simulink model "fft_biplex_test3"  (Simulink 7.6)
settings: Solver=ode45  StartTime=0.0  StopTime=5000  RelTol=1e-3
libraries: xbsIndex_r4 x1382, casper_library x82, monroe_library x27, xps_library x17, dspsigops x16, simulink x1
(part 2 of 13)

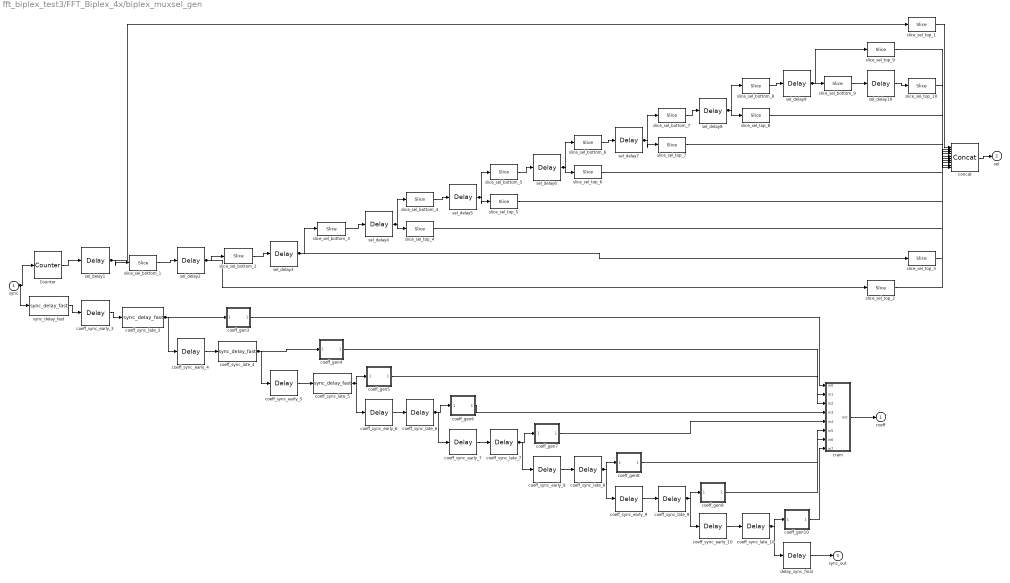
== system fft_biplex_test3/FFT_Biplex_4x/biplex_muxsel_gen ==
  sync : Inport
  Counter : xbsIndex_r4/Counter  cnt_type=Free Running  cnt_to=Inf  operation=Up  start_count=0  cnt_by_val=1  arith_type=Unsigned  n_bits=10  bin_pt=0  load_pin=off  rst=on  en=off  explicit_period=on  period=1  dbl_ovrd=off  use_behavioral_HDL=off  implementation=Fabric  block_type=counter
  coeff_gen10 : Subsystem
  coeff_gen3 : Subsystem
  coeff_gen4 : Subsystem
  coeff_gen5 : Subsystem
  coeff_gen6 : Subsystem
  coeff_gen7 : Subsystem
  coeff_gen8 : Subsystem
  coeff_gen9 : Subsystem
  coeff_sync_early_{4..10} (7 alike) : xbsIndex_r4/Delay  en=off  latency=8  dbl_ovrd=off  reg_retiming=off  block_type=delay
  coeff_sync_early_3 : xbsIndex_r4/Delay  en=off  latency=13  dbl_ovrd=off  reg_retiming=off  block_type=delay
  coeff_sync_late_10 : xbsIndex_r4/Delay  en=off  latency=1  dbl_ovrd=off  reg_retiming=off  block_type=delay
  coeff_sync_late_3 : monroe_library/sync_delay_fast  SystemSampleTime=-1  delay_len=128
  coeff_sync_late_4 : monroe_library/sync_delay_fast  SystemSampleTime=-1  delay_len=64
  coeff_sync_late_5 : monroe_library/sync_delay_fast  SystemSampleTime=-1  delay_len=32
  coeff_sync_late_6 : xbsIndex_r4/Delay  en=off  latency=16  dbl_ovrd=off  reg_retiming=off  block_type=delay
  coeff_sync_late_7 : xbsIndex_r4/Delay  en=off  latency=8  dbl_ovrd=off  reg_retiming=off  block_type=delay
  coeff_sync_late_8 : xbsIndex_r4/Delay  en=off  latency=4  dbl_ovrd=off  reg_retiming=off  block_type=delay
  coeff_sync_late_9 : xbsIndex_r4/Delay  en=off  latency=2  dbl_ovrd=off  reg_retiming=off  block_type=delay
  concat : xbsIndex_r4/Concat  num_inputs=10  dbl_ovrd=off  block_type=concat
  cram : Subsystem
  delay_sync_final : xbsIndex_r4/Delay  en=off  latency=6  dbl_ovrd=off  reg_retiming=off  block_type=delay
  sel_delay1 : xbsIndex_r4/Delay  en=off  latency=1  dbl_ovrd=off  reg_retiming=off  block_type=delay
  sel_delay{4..10} (7 alike) : xbsIndex_r4/Delay  en=off  latency=8  dbl_ovrd=off  reg_retiming=off  block_type=delay
  sel_delay2 : xbsIndex_r4/Delay  en=off  latency=4  dbl_ovrd=off  reg_retiming=off  block_type=delay
  sel_delay3 : xbsIndex_r4/Delay  en=off  latency=7  dbl_ovrd=off  reg_retiming=off  block_type=delay
  slice_sel_bottom_1 : xbsIndex_r4/Slice  nbits=9  boolean_output=off  mode=Lower Bit Location + Width  bit1=0  base1=LSB of Input  bit0=0  base0=LSB of Input  dbl_ovrd=off  block_type=slice
  slice_sel_bottom_2 : xbsIndex_r4/Slice  nbits=8  boolean_output=off  mode=Lower Bit Location + Width  bit1=0  base1=LSB of Input  bit0=0  base0=LSB of Input  dbl_ovrd=off  block_type=slice
  slice_sel_bottom_3 : xbsIndex_r4/Slice  nbits=7  boolean_output=off  mode=Lower Bit Location + Width  bit1=0  base1=LSB of Input  bit0=0  base0=LSB of Input  dbl_ovrd=off  block_type=slice
  slice_sel_bottom_4 : xbsIndex_r4/Slice  nbits=6  boolean_output=off  mode=Lower Bit Location + Width  bit1=0  base1=LSB of Input  bit0=0  base0=LSB of Input  dbl_ovrd=off  block_type=slice
  slice_sel_bottom_5 : xbsIndex_r4/Slice  nbits=5  boolean_output=off  mode=Lower Bit Location + Width  bit1=0  base1=LSB of Input  bit0=0  base0=LSB of Input  dbl_ovrd=off  block_type=slice
  slice_sel_bottom_6 : xbsIndex_r4/Slice  nbits=4  boolean_output=off  mode=Lower Bit Location + Width  bit1=0  base1=LSB of Input  bit0=0  base0=LSB of Input  dbl_ovrd=off  block_type=slice
  slice_sel_bottom_7 : xbsIndex_r4/Slice  nbits=3  boolean_output=off  mode=Lower Bit Location + Width  bit1=0  base1=LSB of Input  bit0=0  base0=LSB of Input  dbl_ovrd=off  block_type=slice
  slice_sel_bottom_8 : xbsIndex_r4/Slice  nbits=2  boolean_output=off  mode=Lower Bit Location + Width  bit1=0  base1=LSB of Input  bit0=0  base0=LSB of Input  dbl_ovrd=off  block_type=slice
  slice_sel_bottom_9 : xbsIndex_r4/Slice  nbits=1  boolean_output=off  mode=Lower Bit Location + Width  bit1=0  base1=LSB of Input  bit0=0  base0=LSB of Input  dbl_ovrd=off  block_type=slice
  slice_sel_top_{1..10} (10 alike) : xbsIndex_r4/Slice  nbits=1  boolean_output=on  mode=Upper Bit Location + Width  bit1=0  base1=MSB of Input  bit0=0  base0=MSB of Input  dbl_ovrd=off  block_type=slice
  sync_delay_fast : monroe_library/sync_delay_fast  SystemSampleTime=-1  delay_len=768
  coeff : Outport
  sel : Outport  Port=2
  sync_out : Outport  Port=3
  wires:
  sync_delay_fast/1 -> coeff_sync_early_3/1
  coeff_sync_early_3/1 -> coeff_sync_late_3/1
  coeff_sync_early_4/1 -> coeff_sync_late_4/1
  coeff_sync_early_5/1 -> coeff_sync_late_5/1
  coeff_sync_early_6/1 -> coeff_sync_late_6/1
  coeff_sync_early_7/1 -> coeff_sync_late_7/1
  coeff_sync_early_8/1 -> coeff_sync_late_8/1
  coeff_sync_early_9/1 -> coeff_sync_late_9/1
  coeff_sync_early_10/1 -> coeff_sync_late_10/1
  coeff_gen3/1(coeff) -> cram/1(in0)
  coeff_gen4/1(coeff) -> cram/2(in1)
  coeff_gen5/1(coeff) -> cram/3(in2)
  coeff_gen6/1(coeff) -> cram/4(in3)
  coeff_gen7/1(coeff) -> cram/5(in4)
  coeff_gen8/1(coeff) -> cram/6(in5)
  coeff_gen9/1(coeff) -> cram/7(in6)
  coeff_gen10/1(coeff) -> cram/8(in7)
  cram/1(out) -> coeff/1
  Counter/1 -> sel_delay1/1
  slice_sel_bottom_1/1 -> sel_delay2/1
  slice_sel_bottom_2/1 -> sel_delay3/1
  slice_sel_bottom_3/1 -> sel_delay4/1
  slice_sel_bottom_4/1 -> sel_delay5/1
  slice_sel_bottom_5/1 -> sel_delay6/1
  slice_sel_bottom_6/1 -> sel_delay7/1
  slice_sel_bottom_7/1 -> sel_delay8/1
  slice_sel_bottom_8/1 -> sel_delay9/1
  slice_sel_bottom_9/1 -> sel_delay10/1
  sel_delay10/1 -> slice_sel_top_10/1
  slice_sel_top_1/1 -> concat/1
  slice_sel_top_2/1 -> concat/2
  slice_sel_top_3/1 -> concat/3
  slice_sel_top_4/1 -> concat/4
  slice_sel_top_5/1 -> concat/5
  slice_sel_top_6/1 -> concat/6
  slice_sel_top_7/1 -> concat/7
  slice_sel_top_8/1 -> concat/8
  slice_sel_top_9/1 -> concat/9
  slice_sel_top_10/1 -> concat/10
  concat/1 -> sel/1
  delay_sync_final/1 -> sync_out/1
  sel_delay9/1 -> slice_sel_top_9/1, slice_sel_bottom_9/1
  sel_delay8/1 -> slice_sel_top_8/1, slice_sel_bottom_8/1
  sel_delay7/1 -> slice_sel_top_7/1, slice_sel_bottom_7/1
  sel_delay6/1 -> slice_sel_top_6/1, slice_sel_bottom_6/1
  sel_delay5/1 -> slice_sel_top_5/1, slice_sel_bottom_5/1
  sel_delay4/1 -> slice_sel_top_4/1, slice_sel_bottom_4/1
  sel_delay3/1 -> slice_sel_top_3/1, slice_sel_bottom_3/1
  sel_delay2/1 -> slice_sel_top_2/1, slice_sel_bottom_2/1
  sel_delay1/1 -> slice_sel_top_1/1, slice_sel_bottom_1/1
  coeff_sync_late_10/1 -> coeff_gen10/1(sync), delay_sync_final/1
  coeff_sync_late_9/1 -> coeff_gen9/1(sync), coeff_sync_early_10/1
  coeff_sync_late_8/1 -> coeff_gen8/1(sync), coeff_sync_early_9/1
  coeff_sync_late_7/1 -> coeff_gen7/1(sync), coeff_sync_early_8/1
  coeff_sync_late_6/1 -> coeff_gen6/1(sync), coeff_sync_early_7/1
  coeff_sync_late_5/1 -> coeff_gen5/1(sync), coeff_sync_early_6/1
  coeff_sync_late_4/1 -> coeff_gen4/1(sync), coeff_sync_early_5/1
  coeff_sync_late_3/1 -> coeff_gen3/1(sync), coeff_sync_early_4/1
  sync/1 -> sync_delay_fast/1, Counter/1

== system fft_biplex_test3/FFT_Biplex_4x/cram0 ==
  in0 : Inport
  in1 : Inport  Port=2
  concat : xbsIndex_r4/Concat  num_inputs=2  dbl_ovrd=off  block_type=concat
  reinterpret_1 : xbsIndex_r4/Reinterpret  force_arith_type=on  arith_type=Unsigned  force_bin_pt=on  bin_pt=0  block_type=reinterpret
      settings: infoedit="Changes signal type without altering the binary representation.   You can changed the signal between signed and unsigned, and relocate the binary point.<br><br>Hardware notes: In hardware this block costs nothing.<br><br>Example:  Suppose the input is 6 bits wide, signed, with 2 fractional bits, and the output is forced to unsigned with 0 fractional bits.  Then an input of -2.0 (1110.00 in binary 2's complement) becomes an output of 56 (111000 in binary)."
  reinterpret_2 : xbsIndex_r4/Reinterpret  force_arith_type=on  arith_type=Unsigned  force_bin_pt=on  bin_pt=0  block_type=reinterpret
      settings: infoedit="Changes signal type without altering the binary representation.   You can changed the signal between signed and unsigned, and relocate the binary point.<br><br>Hardware notes: In hardware this block costs nothing.<br><br>Example:  Suppose the input is 6 bits wide, signed, with 2 fractional bits, and the output is forced to unsigned with 0 fractional bits.  Then an input of -2.0 (1110.00 in binary 2's complement) becomes an output of 56 (111000 in binary)."
  out : Outport
  wires:
  in0/1 -> reinterpret_1/1
  in1/1 -> reinterpret_2/1
  reinterpret_1/1 -> concat/1
  reinterpret_2/1 -> concat/2
  concat/1 -> out/1

== system fft_biplex_test3/FFT_Biplex_4x/cram1 ==
  in0 : Inport
  in1 : Inport  Port=2
  concat : xbsIndex_r4/Concat  num_inputs=2  dbl_ovrd=off  block_type=concat
  reinterpret_1 : xbsIndex_r4/Reinterpret  force_arith_type=on  arith_type=Unsigned  force_bin_pt=on  bin_pt=0  block_type=reinterpret
      settings: infoedit="Changes signal type without altering the binary representation.   You can changed the signal between signed and unsigned, and relocate the binary point.<br><br>Hardware notes: In hardware this block costs nothing.<br><br>Example:  Suppose the input is 6 bits wide, signed, with 2 fractional bits, and the output is forced to unsigned with 0 fractional bits.  Then an input of -2.0 (1110.00 in binary 2's complement) becomes an output of 56 (111000 in binary)."
  reinterpret_2 : xbsIndex_r4/Reinterpret  force_arith_type=on  arith_type=Unsigned  force_bin_pt=on  bin_pt=0  block_type=reinterpret
      settings: infoedit="Changes signal type without altering the binary representation.   You can changed the signal between signed and unsigned, and relocate the binary point.<br><br>Hardware notes: In hardware this block costs nothing.<br><br>Example:  Suppose the input is 6 bits wide, signed, with 2 fractional bits, and the output is forced to unsigned with 0 fractional bits.  Then an input of -2.0 (1110.00 in binary 2's complement) becomes an output of 56 (111000 in binary)."
  out : Outport
  wires:
  in0/1 -> reinterpret_1/1
  in1/1 -> reinterpret_2/1
  reinterpret_1/1 -> concat/1
  reinterpret_2/1 -> concat/2
  concat/1 -> out/1

== system fft_biplex_test3/FFT_Biplex_4x/stage_1 ==
  a : Inport
  b : Inport  Port=2
  sync : Inport  Port=3
  mux_sel : Inport  Port=4
  Mux : xbsIndex_r4/Mux  inputs=2  en=off  latency=0  precision=Full  arith_type="Signed  (2's comp)"  n_bits=8  bin_pt=2  quantization=Truncate  overflow=Wrap  dbl_ovrd=off  block_type=mux
  Mux1 : xbsIndex_r4/Mux  inputs=2  en=off  latency=0  precision=Full  arith_type="Signed  (2's comp)"  n_bits=8  bin_pt=2  quantization=Truncate  overflow=Wrap  dbl_ovrd=off  block_type=mux
  delay_mid : xbsIndex_r4/Delay  en=off  latency=1  dbl_ovrd=off  reg_retiming=off  block_type=delay
  delay_mid1 : xbsIndex_r4/Delay  en=off  latency=1  dbl_ovrd=off  reg_retiming=off  block_type=delay
  delay_start : xbsIndex_r4/Delay  en=off  latency=1  dbl_ovrd=off  reg_retiming=off  block_type=delay
  delay_start1 : xbsIndex_r4/Delay  en=off  latency=1  dbl_ovrd=off  reg_retiming=off  block_type=delay
  double_delay_bram_fast : monroe_library/double_delay_bram_fast  SystemSampleTime=-1  delay_len=512  bram_latency=2  register_counter=0
  sync_delay_fast1 : monroe_library/sync_delay_fast  SystemSampleTime=-1  delay_len=512
  twiddle_stage1 : monroe_library/twiddle_stage1  SystemSampleTime=-1  input_bit_width=18  out_n_bits=18  downshift_at_end=1
  a+bw : Outport
  a-bw : Outport  Port=2
  sync_out : Outport  Port=3
  wires:
  Mux1/1 -> double_delay_bram_fast/1
  double_delay_bram_fast/1 -> delay_mid/1
  Mux/1 -> delay_mid1/1
  a/1 -> delay_start/1
  b/1 -> delay_start1/1
  delay_start1/1 -> double_delay_bram_fast/2
  sync/1 -> sync_delay_fast1/1
  delay_mid/1 -> twiddle_stage1/1
  delay_mid1/1 -> twiddle_stage1/2
  sync_delay_fast1/1 -> twiddle_stage1/3
  twiddle_stage1/1 -> a+bw/1
  twiddle_stage1/2 -> a-bw/1
  twiddle_stage1/3 -> sync_out/1
  delay_start/1 -> Mux/3, Mux1/2
  double_delay_bram_fast/2 -> Mux/2, Mux1/3
  mux_sel/1 -> Mux/1, Mux1/1

== system fft_biplex_test3/FFT_Biplex_4x/stage_10 ==
  a : Inport
  b : Inport  Port=2
  sync : Inport  Port=3
  coeff : Inport  Port=4
  mux_sel : Inport  Port=5
  Mux : xbsIndex_r4/Mux  inputs=2  en=off  latency=0  precision=Full  arith_type="Signed  (2's comp)"  n_bits=8  bin_pt=2  quantization=Truncate  overflow=Wrap  dbl_ovrd=off  block_type=mux
  Mux1 : xbsIndex_r4/Mux  inputs=2  en=off  latency=0  precision=Full  arith_type="Signed  (2's comp)"  n_bits=8  bin_pt=2  quantization=Truncate  overflow=Wrap  dbl_ovrd=off  block_type=mux
  delay_ddbf_1 : xbsIndex_r4/Delay  en=off  latency=1  dbl_ovrd=off  reg_retiming=off  block_type=delay
  delay_ddbf_2 : xbsIndex_r4/Delay  en=off  latency=1  dbl_ovrd=off  reg_retiming=off  block_type=delay
  delay_end : xbsIndex_r4/Delay  en=off  latency=2  dbl_ovrd=off  reg_retiming=off  block_type=delay
  delay_mid : xbsIndex_r4/Delay  en=off  latency=2  dbl_ovrd=off  reg_retiming=off  block_type=delay
  delay_mid1 : xbsIndex_r4/Delay  en=off  latency=1  dbl_ovrd=off  reg_retiming=off  block_type=delay
  delay_start : xbsIndex_r4/Delay  en=off  latency=1  dbl_ovrd=off  reg_retiming=off  block_type=delay
  delay_start1 : xbsIndex_r4/Delay  en=off  latency=1  dbl_ovrd=off  reg_retiming=off  block_type=delay
  sync_delay : xbsIndex_r4/Delay  en=off  latency=1  dbl_ovrd=off  reg_retiming=off  block_type=delay
  twiddle_cheap : monroe_library/twiddle_cheap  SystemSampleTime=-1  a_n_bits=18  a_bin_pt=17  b_n_bits=18  b_bin_pt=17  w_n_bits=18  w_bin_pt=17  a_delay=0  apbw_delay=0  out_n_bits=18  downshift_at_end=1
  a+bw : Outport
  a-bw : Outport  Port=2
  sync_out : Outport  Port=3
  wires:
  Mux1/1 -> delay_ddbf_1/1
  delay_end/1 -> a+bw/1
  delay_ddbf_1/1 -> delay_mid/1
  Mux/1 -> delay_mid1/1
  a/1 -> delay_start/1
  b/1 -> delay_start1/1
  delay_start1/1 -> delay_ddbf_2/1
  sync/1 -> sync_delay/1
  delay_mid/1 -> twiddle_cheap/1
  delay_mid1/1 -> twiddle_cheap/2
  coeff/1 -> twiddle_cheap/3
  sync_delay/1 -> twiddle_cheap/4
  twiddle_cheap/1 -> delay_end/1
  twiddle_cheap/2 -> a-bw/1
  twiddle_cheap/3 -> sync_out/1
  delay_start/1 -> Mux/3, Mux1/2
  delay_ddbf_2/1 -> Mux/2, Mux1/3
  mux_sel/1 -> Mux/1, Mux1/1

== system fft_biplex_test3/FFT_Biplex_4x/stage_2 ==
  a : Inport
  b : Inport  Port=2
  sync : Inport  Port=3
  mux_sel : Inport  Port=4
  Mux : xbsIndex_r4/Mux  inputs=2  en=off  latency=0  precision=Full  arith_type="Signed  (2's comp)"  n_bits=8  bin_pt=2  quantization=Truncate  overflow=Wrap  dbl_ovrd=off  block_type=mux
  Mux1 : xbsIndex_r4/Mux  inputs=2  en=off  latency=0  precision=Full  arith_type="Signed  (2's comp)"  n_bits=8  bin_pt=2  quantization=Truncate  overflow=Wrap  dbl_ovrd=off  block_type=mux
  delay_mid : xbsIndex_r4/Delay  en=off  latency=1  dbl_ovrd=off  reg_retiming=off  block_type=delay
  delay_mid1 : xbsIndex_r4/Delay  en=off  latency=1  dbl_ovrd=off  reg_retiming=off  block_type=delay
  delay_start : xbsIndex_r4/Delay  en=off  latency=1  dbl_ovrd=off  reg_retiming=off  block_type=delay
  delay_start1 : xbsIndex_r4/Delay  en=off  latency=1  dbl_ovrd=off  reg_retiming=off  block_type=delay
  delay_stg2_sel : xbsIndex_r4/Delay  en=off  latency=1  dbl_ovrd=off  reg_retiming=off  block_type=delay
  double_delay_bram_fast : monroe_library/double_delay_bram_fast  SystemSampleTime=-1  delay_len=256  bram_latency=2  register_counter=0
  sync_delay_fast2 : monroe_library/sync_delay_fast  SystemSampleTime=-1  delay_len=256
  twiddle_stage2 : monroe_library/twiddle_stage2  SystemSampleTime=-1  FFTSize=10  input_bit_width=18  out_n_bits=18  downshift_at_end=1
  a+bw : Outport
  a-bw : Outport  Port=2
  sync_out : Outport  Port=3
  wires:
  Mux1/1 -> double_delay_bram_fast/1
  double_delay_bram_fast/1 -> delay_mid/1
  Mux/1 -> delay_mid1/1
  a/1 -> delay_start/1
  b/1 -> delay_start1/1
  delay_start1/1 -> double_delay_bram_fast/2
  sync/1 -> sync_delay_fast2/1
  delay_mid/1 -> twiddle_stage2/1
  delay_mid1/1 -> twiddle_stage2/2
  delay_stg2_sel/1 -> twiddle_stage2/3
  sync_delay_fast2/1 -> twiddle_stage2/4
  twiddle_stage2/1 -> a+bw/1
  twiddle_stage2/2 -> a-bw/1
  twiddle_stage2/3 -> sync_out/1
  delay_start/1 -> Mux/3, Mux1/2
  double_delay_bram_fast/2 -> Mux/2, Mux1/3
  mux_sel/1 -> Mux/1, Mux1/1, delay_stg2_sel/1

== system fft_biplex_test3/FFT_Biplex_4x/stage_3 ==
  a : Inport
  b : Inport  Port=2
  sync : Inport  Port=3
  coeff : Inport  Port=4
  mux_sel : Inport  Port=5
  Mux : xbsIndex_r4/Mux  inputs=2  en=off  latency=0  precision=Full  arith_type="Signed  (2's comp)"  n_bits=8  bin_pt=2  quantization=Truncate  overflow=Wrap  dbl_ovrd=off  block_type=mux
  Mux1 : xbsIndex_r4/Mux  inputs=2  en=off  latency=0  precision=Full  arith_type="Signed  (2's comp)"  n_bits=8  bin_pt=2  quantization=Truncate  overflow=Wrap  dbl_ovrd=off  block_type=mux
  delay_end : xbsIndex_r4/Delay  en=off  latency=2  dbl_ovrd=off  reg_retiming=off  block_type=delay
  delay_mid : xbsIndex_r4/Delay  en=off  latency=2  dbl_ovrd=off  reg_retiming=off  block_type=delay
  delay_mid1 : xbsIndex_r4/Delay  en=off  latency=1  dbl_ovrd=off  reg_retiming=off  block_type=delay
  delay_start : xbsIndex_r4/Delay  en=off  latency=1  dbl_ovrd=off  reg_retiming=off  block_type=delay
  delay_start1 : xbsIndex_r4/Delay  en=off  latency=1  dbl_ovrd=off  reg_retiming=off  block_type=delay
  double_delay_bram_fast : monroe_library/double_delay_bram_fast  SystemSampleTime=-1  delay_len=128  bram_latency=2  register_counter=0
  sync_delay_fast3 : monroe_library/sync_delay_fast  SystemSampleTime=-1  delay_len=128
  twiddle_cheap : monroe_library/twiddle_cheap  SystemSampleTime=-1  a_n_bits=18  a_bin_pt=17  b_n_bits=18  b_bin_pt=17  w_n_bits=18  w_bin_pt=17  a_delay=0  apbw_delay=0  out_n_bits=18  downshift_at_end=1
  a+bw : Outport
  a-bw : Outport  Port=2
  sync_out : Outport  Port=3
  wires:
  Mux1/1 -> double_delay_bram_fast/1
  delay_end/1 -> a+bw/1
  double_delay_bram_fast/1 -> delay_mid/1
  Mux/1 -> delay_mid1/1
  a/1 -> delay_start/1
  b/1 -> delay_start1/1
  delay_start1/1 -> double_delay_bram_fast/2
  sync/1 -> sync_delay_fast3/1
  delay_mid/1 -> twiddle_cheap/1
  delay_mid1/1 -> twiddle_cheap/2
  coeff/1 -> twiddle_cheap/3
  sync_delay_fast3/1 -> twiddle_cheap/4
  twiddle_cheap/1 -> delay_end/1
  twiddle_cheap/2 -> a-bw/1
  twiddle_cheap/3 -> sync_out/1
  delay_start/1 -> Mux/3, Mux1/2
  double_delay_bram_fast/2 -> Mux/2, Mux1/3
  mux_sel/1 -> Mux/1, Mux1/1

== system fft_biplex_test3/FFT_Biplex_4x/stage_4 ==
  a : Inport
  b : Inport  Port=2
  sync : Inport  Port=3
  coeff : Inport  Port=4
  mux_sel : Inport  Port=5
  Mux : xbsIndex_r4/Mux  inputs=2  en=off  latency=0  precision=Full  arith_type="Signed  (2's comp)"  n_bits=8  bin_pt=2  quantization=Truncate  overflow=Wrap  dbl_ovrd=off  block_type=mux
  Mux1 : xbsIndex_r4/Mux  inputs=2  en=off  latency=0  precision=Full  arith_type="Signed  (2's comp)"  n_bits=8  bin_pt=2  quantization=Truncate  overflow=Wrap  dbl_ovrd=off  block_type=mux
  delay_end : xbsIndex_r4/Delay  en=off  latency=2  dbl_ovrd=off  reg_retiming=off  block_type=delay
  delay_mid : xbsIndex_r4/Delay  en=off  latency=2  dbl_ovrd=off  reg_retiming=off  block_type=delay
  delay_mid1 : xbsIndex_r4/Delay  en=off  latency=1  dbl_ovrd=off  reg_retiming=off  block_type=delay
  delay_start : xbsIndex_r4/Delay  en=off  latency=1  dbl_ovrd=off  reg_retiming=off  block_type=delay
  delay_start1 : xbsIndex_r4/Delay  en=off  latency=1  dbl_ovrd=off  reg_retiming=off  block_type=delay
  double_delay_bram_fast : monroe_library/double_delay_bram_fast  SystemSampleTime=-1  delay_len=64  bram_latency=2  register_counter=0
  sync_delay_fast4 : monroe_library/sync_delay_fast  SystemSampleTime=-1  delay_len=64
  twiddle_cheap : monroe_library/twiddle_cheap  SystemSampleTime=-1  a_n_bits=18  a_bin_pt=17  b_n_bits=18  b_bin_pt=17  w_n_bits=18  w_bin_pt=17  a_delay=0  apbw_delay=0  out_n_bits=18  downshift_at_end=1
  a+bw : Outport
  a-bw : Outport  Port=2
  sync_out : Outport  Port=3
  wires:
  Mux1/1 -> double_delay_bram_fast/1
  delay_end/1 -> a+bw/1
  double_delay_bram_fast/1 -> delay_mid/1
  Mux/1 -> delay_mid1/1
  a/1 -> delay_start/1
  b/1 -> delay_start1/1
  delay_start1/1 -> double_delay_bram_fast/2
  sync/1 -> sync_delay_fast4/1
  delay_mid/1 -> twiddle_cheap/1
  delay_mid1/1 -> twiddle_cheap/2
  coeff/1 -> twiddle_cheap/3
  sync_delay_fast4/1 -> twiddle_cheap/4
  twiddle_cheap/1 -> delay_end/1
  twiddle_cheap/2 -> a-bw/1
  twiddle_cheap/3 -> sync_out/1
  delay_start/1 -> Mux/3, Mux1/2
  double_delay_bram_fast/2 -> Mux/2, Mux1/3
  mux_sel/1 -> Mux/1, Mux1/1

== system fft_biplex_test3/FFT_Biplex_4x/stage_5 ==
  a : Inport
  b : Inport  Port=2
  sync : Inport  Port=3
  coeff : Inport  Port=4
  mux_sel : Inport  Port=5
  Mux : xbsIndex_r4/Mux  inputs=2  en=off  latency=0  precision=Full  arith_type="Signed  (2's comp)"  n_bits=8  bin_pt=2  quantization=Truncate  overflow=Wrap  dbl_ovrd=off  block_type=mux
  Mux1 : xbsIndex_r4/Mux  inputs=2  en=off  latency=0  precision=Full  arith_type="Signed  (2's comp)"  n_bits=8  bin_pt=2  quantization=Truncate  overflow=Wrap  dbl_ovrd=off  block_type=mux
  delay_end : xbsIndex_r4/Delay  en=off  latency=2  dbl_ovrd=off  reg_retiming=off  block_type=delay
  delay_mid : xbsIndex_r4/Delay  en=off  latency=2  dbl_ovrd=off  reg_retiming=off  block_type=delay
  delay_mid1 : xbsIndex_r4/Delay  en=off  latency=1  dbl_ovrd=off  reg_retiming=off  block_type=delay
  delay_start : xbsIndex_r4/Delay  en=off  latency=1  dbl_ovrd=off  reg_retiming=off  block_type=delay
  delay_start1 : xbsIndex_r4/Delay  en=off  latency=1  dbl_ovrd=off  reg_retiming=off  block_type=delay
  double_delay_bram_fast : monroe_library/double_delay_bram_fast  SystemSampleTime=-1  delay_len=32  bram_latency=2  register_counter=0
  sync_delay_fast5 : monroe_library/sync_delay_fast  SystemSampleTime=-1  delay_len=32
  twiddle_cheap : monroe_library/twiddle_cheap  SystemSampleTime=-1  a_n_bits=18  a_bin_pt=17  b_n_bits=18  b_bin_pt=17  w_n_bits=18  w_bin_pt=17  a_delay=0  apbw_delay=0  out_n_bits=18  downshift_at_end=1
  a+bw : Outport
  a-bw : Outport  Port=2
  sync_out : Outport  Port=3
  wires:
  Mux1/1 -> double_delay_bram_fast/1
  delay_end/1 -> a+bw/1
  double_delay_bram_fast/1 -> delay_mid/1
  Mux/1 -> delay_mid1/1
  a/1 -> delay_start/1
  b/1 -> delay_start1/1
  delay_start1/1 -> double_delay_bram_fast/2
  sync/1 -> sync_delay_fast5/1
  delay_mid/1 -> twiddle_cheap/1
  delay_mid1/1 -> twiddle_cheap/2
  coeff/1 -> twiddle_cheap/3
  sync_delay_fast5/1 -> twiddle_cheap/4
  twiddle_cheap/1 -> delay_end/1
  twiddle_cheap/2 -> a-bw/1
  twiddle_cheap/3 -> sync_out/1
  delay_start/1 -> Mux/3, Mux1/2
  double_delay_bram_fast/2 -> Mux/2, Mux1/3
  mux_sel/1 -> Mux/1, Mux1/1

== system fft_biplex_test3/FFT_Biplex_4x/stage_6 ==
  a : Inport
  b : Inport  Port=2
  sync : Inport  Port=3
  coeff : Inport  Port=4
  mux_sel : Inport  Port=5
  Mux : xbsIndex_r4/Mux  inputs=2  en=off  latency=0  precision=Full  arith_type="Signed  (2's comp)"  n_bits=8  bin_pt=2  quantization=Truncate  overflow=Wrap  dbl_ovrd=off  block_type=mux
  Mux1 : xbsIndex_r4/Mux  inputs=2  en=off  latency=0  precision=Full  arith_type="Signed  (2's comp)"  n_bits=8  bin_pt=2  quantization=Truncate  overflow=Wrap  dbl_ovrd=off  block_type=mux
  delay_ddbf_1 : xbsIndex_r4/Delay  en=off  latency=16  dbl_ovrd=off  reg_retiming=off  block_type=delay
  delay_ddbf_2 : xbsIndex_r4/Delay  en=off  latency=16  dbl_ovrd=off  reg_retiming=off  block_type=delay
  delay_end : xbsIndex_r4/Delay  en=off  latency=2  dbl_ovrd=off  reg_retiming=off  block_type=delay
  delay_mid : xbsIndex_r4/Delay  en=off  latency=2  dbl_ovrd=off  reg_retiming=off  block_type=delay
  delay_mid1 : xbsIndex_r4/Delay  en=off  latency=1  dbl_ovrd=off  reg_retiming=off  block_type=delay
  delay_start : xbsIndex_r4/Delay  en=off  latency=1  dbl_ovrd=off  reg_retiming=off  block_type=delay
  delay_start1 : xbsIndex_r4/Delay  en=off  latency=1  dbl_ovrd=off  reg_retiming=off  block_type=delay
  sync_delay : xbsIndex_r4/Delay  en=off  latency=16  dbl_ovrd=off  reg_retiming=off  block_type=delay
  twiddle_cheap : monroe_library/twiddle_cheap  SystemSampleTime=-1  a_n_bits=18  a_bin_pt=17  b_n_bits=18  b_bin_pt=17  w_n_bits=18  w_bin_pt=17  a_delay=0  apbw_delay=0  out_n_bits=18  downshift_at_end=1
  a+bw : Outport
  a-bw : Outport  Port=2
  sync_out : Outport  Port=3
  wires:
  Mux1/1 -> delay_ddbf_1/1
  delay_end/1 -> a+bw/1
  delay_ddbf_1/1 -> delay_mid/1
  Mux/1 -> delay_mid1/1
  a/1 -> delay_start/1
  b/1 -> delay_start1/1
  delay_start1/1 -> delay_ddbf_2/1
  sync/1 -> sync_delay/1
  delay_mid/1 -> twiddle_cheap/1
  delay_mid1/1 -> twiddle_cheap/2
  coeff/1 -> twiddle_cheap/3
  sync_delay/1 -> twiddle_cheap/4
  twiddle_cheap/1 -> delay_end/1
  twiddle_cheap/2 -> a-bw/1
  twiddle_cheap/3 -> sync_out/1
  delay_start/1 -> Mux/3, Mux1/2
  delay_ddbf_2/1 -> Mux/2, Mux1/3
  mux_sel/1 -> Mux/1, Mux1/1

== system fft_biplex_test3/FFT_Biplex_4x/stage_7 ==
  a : Inport
  b : Inport  Port=2
  sync : Inport  Port=3
  coeff : Inport  Port=4
  mux_sel : Inport  Port=5
  Mux : xbsIndex_r4/Mux  inputs=2  en=off  latency=0  precision=Full  arith_type="Signed  (2's comp)"  n_bits=8  bin_pt=2  quantization=Truncate  overflow=Wrap  dbl_ovrd=off  block_type=mux
  Mux1 : xbsIndex_r4/Mux  inputs=2  en=off  latency=0  precision=Full  arith_type="Signed  (2's comp)"  n_bits=8  bin_pt=2  quantization=Truncate  overflow=Wrap  dbl_ovrd=off  block_type=mux
  delay_ddbf_1 : xbsIndex_r4/Delay  en=off  latency=8  dbl_ovrd=off  reg_retiming=off  block_type=delay
  delay_ddbf_2 : xbsIndex_r4/Delay  en=off  latency=8  dbl_ovrd=off  reg_retiming=off  block_type=delay
  delay_end : xbsIndex_r4/Delay  en=off  latency=2  dbl_ovrd=off  reg_retiming=off  block_type=delay
  delay_mid : xbsIndex_r4/Delay  en=off  latency=2  dbl_ovrd=off  reg_retiming=off  block_type=delay
  delay_mid1 : xbsIndex_r4/Delay  en=off  latency=1  dbl_ovrd=off  reg_retiming=off  block_type=delay
  delay_start : xbsIndex_r4/Delay  en=off  latency=1  dbl_ovrd=off  reg_retiming=off  block_type=delay
  delay_start1 : xbsIndex_r4/Delay  en=off  latency=1  dbl_ovrd=off  reg_retiming=off  block_type=delay
  sync_delay : xbsIndex_r4/Delay  en=off  latency=8  dbl_ovrd=off  reg_retiming=off  block_type=delay
  twiddle_cheap : monroe_library/twiddle_cheap  SystemSampleTime=-1  a_n_bits=18  a_bin_pt=17  b_n_bits=18  b_bin_pt=17  w_n_bits=18  w_bin_pt=17  a_delay=0  apbw_delay=0  out_n_bits=18  downshift_at_end=1
  a+bw : Outport
  a-bw : Outport  Port=2
  sync_out : Outport  Port=3
  wires:
  Mux1/1 -> delay_ddbf_1/1
  delay_end/1 -> a+bw/1
  delay_ddbf_1/1 -> delay_mid/1
  Mux/1 -> delay_mid1/1
  a/1 -> delay_start/1
  b/1 -> delay_start1/1
  delay_start1/1 -> delay_ddbf_2/1
  sync/1 -> sync_delay/1
  delay_mid/1 -> twiddle_cheap/1
  delay_mid1/1 -> twiddle_cheap/2
  coeff/1 -> twiddle_cheap/3
  sync_delay/1 -> twiddle_cheap/4
  twiddle_cheap/1 -> delay_end/1
  twiddle_cheap/2 -> a-bw/1
  twiddle_cheap/3 -> sync_out/1
  delay_start/1 -> Mux/3, Mux1/2
  delay_ddbf_2/1 -> Mux/2, Mux1/3
  mux_sel/1 -> Mux/1, Mux1/1

== system fft_biplex_test3/FFT_Biplex_4x/stage_8 ==
  a : Inport
  b : Inport  Port=2
  sync : Inport  Port=3
  coeff : Inport  Port=4
  mux_sel : Inport  Port=5
  Mux : xbsIndex_r4/Mux  inputs=2  en=off  latency=0  precision=Full  arith_type="Signed  (2's comp)"  n_bits=8  bin_pt=2  quantization=Truncate  overflow=Wrap  dbl_ovrd=off  block_type=mux
  Mux1 : xbsIndex_r4/Mux  inputs=2  en=off  latency=0  precision=Full  arith_type="Signed  (2's comp)"  n_bits=8  bin_pt=2  quantization=Truncate  overflow=Wrap  dbl_ovrd=off  block_type=mux
  delay_ddbf_1 : xbsIndex_r4/Delay  en=off  latency=4  dbl_ovrd=off  reg_retiming=off  block_type=delay
  delay_ddbf_2 : xbsIndex_r4/Delay  en=off  latency=4  dbl_ovrd=off  reg_retiming=off  block_type=delay
  delay_end : xbsIndex_r4/Delay  en=off  latency=2  dbl_ovrd=off  reg_retiming=off  block_type=delay
  delay_mid : xbsIndex_r4/Delay  en=off  latency=2  dbl_ovrd=off  reg_retiming=off  block_type=delay
  delay_mid1 : xbsIndex_r4/Delay  en=off  latency=1  dbl_ovrd=off  reg_retiming=off  block_type=delay
  delay_start : xbsIndex_r4/Delay  en=off  latency=1  dbl_ovrd=off  reg_retiming=off  block_type=delay
  delay_start1 : xbsIndex_r4/Delay  en=off  latency=1  dbl_ovrd=off  reg_retiming=off  block_type=delay
  sync_delay : xbsIndex_r4/Delay  en=off  latency=4  dbl_ovrd=off  reg_retiming=off  block_type=delay
  twiddle_cheap : monroe_library/twiddle_cheap  SystemSampleTime=-1  a_n_bits=18  a_bin_pt=17  b_n_bits=18  b_bin_pt=17  w_n_bits=18  w_bin_pt=17  a_delay=0  apbw_delay=0  out_n_bits=18  downshift_at_end=1
  a+bw : Outport
  a-bw : Outport  Port=2
  sync_out : Outport  Port=3
  wires:
  Mux1/1 -> delay_ddbf_1/1
  delay_end/1 -> a+bw/1
  delay_ddbf_1/1 -> delay_mid/1
  Mux/1 -> delay_mid1/1
  a/1 -> delay_start/1
  b/1 -> delay_start1/1
  delay_start1/1 -> delay_ddbf_2/1
  sync/1 -> sync_delay/1
  delay_mid/1 -> twiddle_cheap/1
  delay_mid1/1 -> twiddle_cheap/2
  coeff/1 -> twiddle_cheap/3
  sync_delay/1 -> twiddle_cheap/4
  twiddle_cheap/1 -> delay_end/1
  twiddle_cheap/2 -> a-bw/1
  twiddle_cheap/3 -> sync_out/1
  delay_start/1 -> Mux/3, Mux1/2
  delay_ddbf_2/1 -> Mux/2, Mux1/3
  mux_sel/1 -> Mux/1, Mux1/1

== system fft_biplex_test3/FFT_Biplex_4x/stage_9 ==
  a : Inport
  b : Inport  Port=2
  sync : Inport  Port=3
  coeff : Inport  Port=4
  mux_sel : Inport  Port=5
  Mux : xbsIndex_r4/Mux  inputs=2  en=off  latency=0  precision=Full  arith_type="Signed  (2's comp)"  n_bits=8  bin_pt=2  quantization=Truncate  overflow=Wrap  dbl_ovrd=off  block_type=mux
  Mux1 : xbsIndex_r4/Mux  inputs=2  en=off  latency=0  precision=Full  arith_type="Signed  (2's comp)"  n_bits=8  bin_pt=2  quantization=Truncate  overflow=Wrap  dbl_ovrd=off  block_type=mux
  delay_ddbf_1 : xbsIndex_r4/Delay  en=off  latency=2  dbl_ovrd=off  reg_retiming=off  block_type=delay
  delay_ddbf_2 : xbsIndex_r4/Delay  en=off  latency=2  dbl_ovrd=off  reg_retiming=off  block_type=delay
  delay_end : xbsIndex_r4/Delay  en=off  latency=2  dbl_ovrd=off  reg_retiming=off  block_type=delay
  delay_mid : xbsIndex_r4/Delay  en=off  latency=2  dbl_ovrd=off  reg_retiming=off  block_type=delay
  delay_mid1 : xbsIndex_r4/Delay  en=off  latency=1  dbl_ovrd=off  reg_retiming=off  block_type=delay
  delay_start : xbsIndex_r4/Delay  en=off  latency=1  dbl_ovrd=off  reg_retiming=off  block_type=delay
  delay_start1 : xbsIndex_r4/Delay  en=off  latency=1  dbl_ovrd=off  reg_retiming=off  block_type=delay
  sync_delay : xbsIndex_r4/Delay  en=off  latency=2  dbl_ovrd=off  reg_retiming=off  block_type=delay
  twiddle_cheap : monroe_library/twiddle_cheap  SystemSampleTime=-1  a_n_bits=18  a_bin_pt=17  b_n_bits=18  b_bin_pt=17  w_n_bits=18  w_bin_pt=17  a_delay=0  apbw_delay=0  out_n_bits=18  downshift_at_end=1
  a+bw : Outport
  a-bw : Outport  Port=2
  sync_out : Outport  Port=3
  wires:
  Mux1/1 -> delay_ddbf_1/1
  delay_end/1 -> a+bw/1
  delay_ddbf_1/1 -> delay_mid/1
  Mux/1 -> delay_mid1/1
  a/1 -> delay_start/1
  b/1 -> delay_start1/1
  delay_start1/1 -> delay_ddbf_2/1
  sync/1 -> sync_delay/1
  delay_mid/1 -> twiddle_cheap/1
  delay_mid1/1 -> twiddle_cheap/2
  coeff/1 -> twiddle_cheap/3
  sync_delay/1 -> twiddle_cheap/4
  twiddle_cheap/1 -> delay_end/1
  twiddle_cheap/2 -> a-bw/1
  twiddle_cheap/3 -> sync_out/1
  delay_start/1 -> Mux/3, Mux1/2
  delay_ddbf_2/1 -> Mux/2, Mux1/3
  mux_sel/1 -> Mux/1, Mux1/1

== system fft_biplex_test3/adc083000x2/adc_sim ==
  sim_adc_data_in : Inport
  adc_bias : Bias  Bias=128  SaturateOnIntegerOverflow=on
  adc_gain : Gain  Gain=128
  overflow_detector : Subsystem  AncestorBlock=casper_library/Misc/of_detect_bus  mask(of_detect_bus){nStreams=16, bit_width=8}
      mask prompts: nStreams "Number of Streams"; bit_width "Bit Width"
      mask init:
      | adc_overflow_detector_init(gcb, ...
      |     'nStreams', nStreams, ...
      |     'bit_width', bit_width);
  sample0_ds : dspsigops/Downsample  N=16  phase=1  InputProcessing=Inherited (this choice will be removed - see release notes)  RateOptions=Enforce single-rate processing  smode=Force single rate  fmode=Maintain input frame size  ic=0
  sample10_ds : dspsigops/Downsample  N=16  phase=11  InputProcessing=Inherited (this choice will be removed - see release notes)  RateOptions=Enforce single-rate processing  smode=Force single rate  fmode=Maintain input frame size  ic=0
  sample11_ds : dspsigops/Downsample  N=16  phase=12  InputProcessing=Inherited (this choice will be removed - see release notes)  RateOptions=Enforce single-rate processing  smode=Force single rate  fmode=Maintain input frame size  ic=0
  sample12_ds : dspsigops/Downsample  N=16  phase=13  InputProcessing=Inherited (this choice will be removed - see release notes)  RateOptions=Enforce single-rate processing  smode=Force single rate  fmode=Maintain input frame size  ic=0
  sample13_ds : dspsigops/Downsample  N=16  phase=14  InputProcessing=Inherited (this choice will be removed - see release notes)  RateOptions=Enforce single-rate processing  smode=Force single rate  fmode=Maintain input frame size  ic=0
  sample14_ds : dspsigops/Downsample  N=16  phase=15  InputProcessing=Inherited (this choice will be removed - see release notes)  RateOptions=Enforce single-rate processing  smode=Force single rate  fmode=Maintain input frame size  ic=0
  sample15_ds : dspsigops/Downsample  N=16  phase=0  InputProcessing=Inherited (this choice will be removed - see release notes)  RateOptions=Enforce single-rate processing  smode=Force single rate  fmode=Maintain input frame size  ic=0
  sample1_ds : dspsigops/Downsample  N=16  phase=2  InputProcessing=Inherited (this choice will be removed - see release notes)  RateOptions=Enforce single-rate processing  smode=Force single rate  fmode=Maintain input frame size  ic=0
  sample2_ds : dspsigops/Downsample  N=16  phase=3  InputProcessing=Inherited (this choice will be removed - see release notes)  RateOptions=Enforce single-rate processing  smode=Force single rate  fmode=Maintain input frame size  ic=0
  sample3_ds : dspsigops/Downsample  N=16  phase=4  InputProcessing=Inherited (this choice will be removed - see release notes)  RateOptions=Enforce single-rate processing  smode=Force single rate  fmode=Maintain input frame size  ic=0
  sample4_ds : dspsigops/Downsample  N=16  phase=5  InputProcessing=Inherited (this choice will be removed - see release notes)  RateOptions=Enforce single-rate processing  smode=Force single rate  fmode=Maintain input frame size  ic=0
  sample5_ds : dspsigops/Downsample  N=16  phase=6  InputProcessing=Inherited (this choice will be removed - see release notes)  RateOptions=Enforce single-rate processing  smode=Force single rate  fmode=Maintain input frame size  ic=0
  sample6_ds : dspsigops/Downsample  N=16  phase=7  InputProcessing=Inherited (this choice will be removed - see release notes)  RateOptions=Enforce single-rate processing  smode=Force single rate  fmode=Maintain input frame size  ic=0
  sample7_ds : dspsigops/Downsample  N=16  phase=8  InputProcessing=Inherited (this choice will be removed - see release notes)  RateOptions=Enforce single-rate processing  smode=Force single rate  fmode=Maintain input frame size  ic=0
  sample8_ds : dspsigops/Downsample  N=16  phase=9  InputProcessing=Inherited (this choice will be removed - see release notes)  RateOptions=Enforce single-rate processing  smode=Force single rate  fmode=Maintain input frame size  ic=0
  sample9_ds : dspsigops/Downsample  N=16  phase=10  InputProcessing=Inherited (this choice will be removed - see release notes)  RateOptions=Enforce single-rate processing  smode=Force single rate  fmode=Maintain input frame size  ic=0
  s0 : Outport
  s1 : Outport  Port=2
  s2 : Outport  Port=3
  s3 : Outport  Port=4
  s4 : Outport  Port=5
  s5 : Outport  Port=6
  s6 : Outport  Port=7
  s7 : Outport  Port=8
  s8 : Outport  Port=9
  s9 : Outport  Port=10
  s10 : Outport  Port=11
  s11 : Outport  Port=12
  s12 : Outport  Port=13
  s13 : Outport  Port=14
  s14 : Outport  Port=15
  s15 : Outport  Port=16
  of : Outport  Port=17
  wires:
  sample15_ds/1 -> s15/1, overflow_detector/16(s15)
  sample14_ds/1 -> s14/1, overflow_detector/15(s14)
  sample13_ds/1 -> s13/1, overflow_detector/14(s13)
  sample12_ds/1 -> s12/1, overflow_detector/13(s12)
  sample11_ds/1 -> s11/1, overflow_detector/12(s11)
  sample10_ds/1 -> s10/1, overflow_detector/11(s10)
  sample9_ds/1 -> s9/1, overflow_detector/10(s9)
  sample8_ds/1 -> s8/1, overflow_detector/9(s8)
  sample7_ds/1 -> s7/1, overflow_detector/8(s7)
  sample6_ds/1 -> s6/1, overflow_detector/7(s6)
  sample5_ds/1 -> s5/1, overflow_detector/6(s5)
  sample4_ds/1 -> s4/1, overflow_detector/5(s4)
  sample3_ds/1 -> s3/1, overflow_detector/4(s3)
  sample2_ds/1 -> s2/1, overflow_detector/3(s2)
  sample1_ds/1 -> s1/1, overflow_detector/2(s1)
  sample0_ds/1 -> s0/1, overflow_detector/1(s0)
  adc_bias/1 -> sample15_ds/1, sample14_ds/1, sample13_ds/1, sample12_ds/1, sample11_ds/1, sample10_ds/1, sample9_ds/1, sample8_ds/1, sample7_ds/1, sample6_ds/1, sample5_ds/1, sample4_ds/1, sample3_ds/1, sample2_ds/1, sample1_ds/1, sample0_ds/1
  overflow_detector/1(overflow) -> of/1
  adc_gain/1 -> adc_bias/1
  sim_adc_data_in/1 -> adc_gain/1
